simulink model "Symmetric"  (R2018a)
settings: Solver=VariableStepAuto  StartTime=0.0  StopTime=0.001  RelTol=1e-3
undefined symbols (not defined in the file or in its folder): fdesignblkfcn, G1, G2, G3, G4, G5, G6, G7, G8, gcbh, get, T
libraries: dspsrcs4 x1, dspxfrm3 x1, dspobslib x1
(part 2 of 2)

== system Symmetric/Filter Bank /Filter 7/Bandpass Filter ==
  In : Inport
  Generated Filter Block : DiscreteFir  Tag=BlockMethodSubSystem  Coefficients=[0.00857375745233986825 -0.0262726370509678599 -0.00974647616296401773 -0.00439060024736811268 0.00283263673597632885 -0.00300721003000267066 -6.2733861075844427e-05 0.00296135556060779037 -0.00404500810835179032 0.00223751069246359239 0.00138756604038855536 -0.00436312984074752833 0.00442339639727916487 -0.00121770484220593369 -0.00320512214454504512 0.00568093053665862796 -0.00419610981840044979 -0.000482360310534853836 0.00514145590278858918 -0.0063507955543423613 0.00303488452209107465 0.00260078232559330389 -0.00654982989014639069 0.00590897293534065841 -0.00108486058876781921 -0.0044740193974794366 0.00679351841095432538 -0.00431977405330382768 -0.00101055174584457636 0.005283664339711505 -0.00560672550614138392 0.00211451149186762466 0.0023205741112376139 -0.00451799441799459987 0.00333453222499137522 -0.000280734646955920516 -0.00206837752446509607 0.00225416836150129155 -0.000913651700026251834 -0.000183799251151528509 2.79031376706901457e-05 0.000711860730427829038 -0.000487077424696307946 -0.0012776694998413809 0.00324488065567231886 -0.00314034683122965371 -4.24935311660271741e-06 0.00441236008519720318 -0.00652422445043266026 0.00385255637203440202 0.00251637322430788707 -0.00814971160958483445 0.00843027333235982744 -0.00234352166622425404 -0.00620099220143535863 0.0109428163666879484 -0.0080137009368117882 -0.000901555730674943033 0.00948326631461534481 -0.011446096708088601 0.00531599608033400499 0.00442367643753116459 -0.0107107510793313029 0.0092538223716912716 -0.0016172246715166652 -0.00626106036570885528 0.00882685050909009887 -0.00509622448983353474 -0.0010741399943965974 0.00476343053662749236 -0.00406196364356412563 0.00108184682714144889 0.00057207759551576164 0.000456313077468849606 -0.00184754756202802368 0.000318960947085945227 0.00437708856474283009 -0.00827631679113341977 0.00617832281311445856 0.0029847507334840543 -0.0134346583353167487 0.016127400067828309 -0.00614861054646659039 -0.0116730422964640528 0.0244821936184197071 -0.0207455194435129039 4.44597263896157333e-06 0.0244893503457132324 -0.0341914771280653271 0.0193444362547145823 0.0121595441397046432 -0.0384022521195573202 0.0389908985431173111 -0.0106923575821091035 -0.028094118131374371 0.0495187699533457815 -0.0363451357813906195 -0.00415963938342176452 0.044069468532439815 -0.0542339770466458287 0.0258413300070809322 0.022164736386769246 -0.0558491959765245252 0.050611147820193457 -0.00935857651434154718 -0.0390234066028688487 0.0601797118853347468 -0.0390234066028688487 -0.00935857651434154718 0.050611147820193457 -0.0558491959765245252 0.022164736386769246 0.0258413300070809322 -0.0542339770466458287 0.044069468532439815 -0.00415963938342176452 -0.0363451357813906195 0.0495187699533457815 -0.028094118131374371 -0.0106923575821091035 0.0389908985431173111 -0.0384022521195573202 0.0121595441397046432 0.0193444362547145823 -0.0341914771280653271 0.0244893503457132324 4.44597263896157333e-06 -0.0207455194435129039 0.0244821936184197071 -0.0116730422964640528 -0.00614861054646659039 0.016127400067828309 -0.0134346583353167487 0.0029847507334840543 0.00617832281311445856 -0.00827631679113341977 0.00437708856474283009 0.000318960947085945227 -0.00184754756202802368 0.000456313077468849606 0.00057207759551576164 0.00108184682714144889 -0.00406196364356412563 0.00476343053662749236 -0.0010741399943965974 -0.00509622448983353474 0.00882685050909009887 -0.00626106036570885528 -0.0016172246715166652 0.0092538223716912716 -0.0107107510793313029 0.00442367643753116459 0.00531599608033400499 -0.011446096708088601 0.00948326631461534481 -0.000901555730674943033 -0.0080137009368117882 0.0109428163666879484 -0.00620099220143535863 -0.00234352166622425404 0.00843027333235982744 -0.00814971160958483445 0.00251637322430788707 0.00385255637203440202 -0.00652422445043266026 0.00441236008519720318 -4.24935311660271741e-06 -0.00314034683122965371 0.00324488065567231886 -0.0012776694998413809 -0.000487077424696307946 0.000711860730427829038 ...(+965 chars)]  InputProcessing=Columns as channels (frame based)
  Out : Outport
  wires:
  In/1 -> Generated Filter Block/1
  Generated Filter Block/1 -> Out/1

== system Symmetric/Filter Bank /Filter 8/Bandpass Filter ==
  In : Inport
  Generated Filter Block : DiscreteFir  Tag=BlockMethodSubSystem  Coefficients=[-0.0251791761247325829 -0.0102217576550982514 0.00641945090901670581 -0.00334354163827728411 0.00185213720214450102 -0.00220643402249874956 0.0039174982369860516 -0.00591114357840174642 0.00694248727990195817 -0.00615618376626782086 0.00354039053172731542 -2.74576649316574658e-05 -0.00286600194798258476 0.003747019727223072 -0.0020873364370468479 -0.00140275635090877514 0.0050148908778130533 -0.00683880809345403535 0.00574601468845681741 -0.00204351944101153647 -0.00259086277759661881 0.00590622375724306464 -0.006224699887651443 0.00334149571420841712 0.0013245637475120095 -0.00544120310683285802 0.00696594009065848625 -0.00519991362844829472 0.00112986032444797966 0.00313543242236372305 -0.00551268772008747278 0.0050274299737679308 -0.00224489946878606668 -0.00115027504636510476 0.00339413409657343896 -0.00356601457704190054 0.00212177296532830217 -0.000169642424935544176 -0.000891487134245472863 0.000756353009021231652 -1.6638269009578887e-05 -0.000307870779907929598 -0.000465532883611990272 0.00205215254009714302 -0.00323864794459314187 0.00269300148977304069 -5.61455369923121995e-06 -0.0037752753920779372 0.00654259626882524106 -0.00631136942372411466 0.00251935660473366152 0.00337002595248607614 -0.00842459339019489654 0.00975817375154321154 -0.00620022665074001361 -0.000856717615039965467 0.0080038780011481396 -0.0115458134242847257 0.00950240262381111048 -0.00276189871061736274 -0.00531566260590729447 0.0106703014710552366 -0.0107111732068328191 0.00567145569636271461 0.00160200286651443241 -0.00730571815386255735 0.00880619588950202689 -0.00598624515496137734 0.00106407781754691393 0.00292125014245447987 -0.00406014819122739543 0.00259187754715095673 -0.000563792716331256924 9.93934293738705263e-05 -0.00183714440444857617 0.00417331784128369913 -0.00437947248985956321 0.00065096006388265504 0.00616305208628449477 -0.0123995003853002491 0.0134349852373020946 -0.00667769571533687739 -0.00614577308337781701 0.0190389122724875307 -0.0244934152161555389 0.0177163012296234143 -3.96529037680604142e-06 -0.0209086768294740738 0.0341936702484474594 -0.0315467951934389687 0.0121507404474161668 0.015910054376491907 -0.0389797478058401189 0.0445624335496773716 -0.0280984986816106633 -0.00389792955641649194 0.0363493203352199049 -0.052847621817576601 0.0440731193557385437 -0.0130281836346955188 -0.0258394733635318903 0.0534981739114132257 -0.0558475191049585401 0.0310194260879065424 0.00935758863050048344 -0.0456895344379586246 0.0601841279737592855 -0.0456895344379586246 0.00935758863050048344 0.0310194260879065424 -0.0558475191049585401 0.0534981739114132257 -0.0258394733635318903 -0.0130281836346955188 0.0440731193557385437 -0.052847621817576601 0.0363493203352199049 -0.00389792955641649194 -0.0280984986816106633 0.0445624335496773716 -0.0389797478058401189 0.015910054376491907 0.0121507404474161668 -0.0315467951934389687 0.0341936702484474594 -0.0209086768294740738 -3.96529037680604142e-06 0.0177163012296234143 -0.0244934152161555389 0.0190389122724875307 -0.00614577308337781701 -0.00667769571533687739 0.0134349852373020946 -0.0123995003853002491 0.00616305208628449477 0.00065096006388265504 -0.00437947248985956321 0.00417331784128369913 -0.00183714440444857617 9.93934293738705263e-05 -0.000563792716331256924 0.00259187754715095673 -0.00406014819122739543 0.00292125014245447987 0.00106407781754691393 -0.00598624515496137734 0.00880619588950202689 -0.00730571815386255735 0.00160200286651443241 0.00567145569636271461 -0.0107111732068328191 0.0106703014710552366 -0.00531566260590729447 -0.00276189871061736274 0.00950240262381111048 -0.0115458134242847257 0.0080038780011481396 -0.000856717615039965467 -0.00620022665074001361 0.00975817375154321154 -0.00842459339019489654 0.00337002595248607614 0.00251935660473366152 -0.00631136942372411466 0.00654259626882524106 -0.0037752753920779372 -5.61455369923121995e-06 0.00269300148977304069 -0.00323864794459314187 0.00205215254009714302 -0.000465532883611990272 -0.000307870779907929598 ...(+959 chars)]  InputProcessing=Columns as channels (frame based)
  Out : Outport
  wires:
  In/1 -> Generated Filter Block/1
  Generated Filter Block/1 -> Out/1
